simulink model "simcape_real_time_V3"  (R2022b)
settings: Solver=FixedStepAuto  StartTime=0.0  StopTime=100  FixedStep=0.002  RelTol=1e-3
undefined symbols (not defined in the file): drone_leg, K_LQR_GOC, pitch_init, roll_init, v_pitch_init, v_roll_init, v_x_init, v_y_init, v_yaw_init, v_z_init, X, x_init, Y, y_init, yaw_init, Z, z_init
libraries: sm_lib x70, nesl_utility x11, simulink x6
(part 4 of 4)

== matlab function simcape_real_time_V3/MATLAB Function ==
  data: T1 input; x2dot output; T2 input; T3 input; T4 input; roll input; pitch input; yaw input; roll_dot input; pitch_dot input; yaw_dot input; y2dot output; z2dot output; roll2dot output; pitch2dot output; yaw2dot output; HS_MSKK input; x_dot input; y_dot input; z_dot input
function [x2dot,y2dot,z2dot,roll2dot,pitch2dot,yaw2dot]= fcn(T1,T2,T3,T4,roll,pitch,yaw,roll_dot,pitch_dot,yaw_dot,HS_MSKK,x_dot,y_dot,z_dot)
    m = 1.7; %kg
    l = 0.25; %m
    % % b = 4.74E-5;
    % % d = 2.35E-7;
    g = 9.81; %ms2
    % % to = 0.05; %Nm
    Ix = 0.0030842; %kg.m2
    Iy = 0.0030842; %kg.m2
    Iz = 0.0032315; %kg.m2
    % Ir = 1E-4; %kg.m2
    U1 = T1+T2+T3+T4;
    U2 = l*(T2-T4);
    U3 = l*(T3-T1);
    U4 = T1-T2+T3-T4;

    x2dot=(U1*(sin(roll)*sin(yaw) + cos(roll)*cos(yaw)*sin(pitch)))/m;
    y2dot=-(U1*(cos(yaw)*sin(roll) - cos(roll)*sin(pitch)*sin(yaw)))/m;
    z2dot=(U1*cos(pitch)*cos(roll))/m - g;
    roll2dot=(Iy*pitch_dot*yaw_dot - Iz*pitch_dot*yaw_dot)/Ix + U2/Ix;
    pitch2dot=U3/Iy + (-Ix*roll_dot*yaw_dot + Iz*roll_dot*yaw_dot)/Iy;
    yaw2dot=U4/Iz + (Ix*pitch_dot*roll_dot - Iy*pitch_dot*roll_dot)/Iz;

% %% Gia lap ma sat theo cong thuc ma sat tuyen tinh voi he so cho truoc la
    FX_Friction     =  -  HS_MSKK * x_dot;
    FY_Friction     =  -  HS_MSKK * y_dot;
    FZ_Friction     =  -  HS_MSKK * z_dot;
    FR_Friction     =  -  HS_MSKK * roll_dot;
    FP_Friction     =  -  HS_MSKK * pitch_dot;
    FYaw_Friction   =  -  HS_MSKK * yaw_dot;
    FX_Limit        =     HS_MSKK /10;
    FY_Limit        =     HS_MSKK /10;
    FZ_Limit        =     HS_MSKK /10;
    FR_Limit        =     HS_MSKK /10;
    FP_Limit        =     HS_MSKK /10;
    FYaw_Limit      =     HS_MSKK /10;
    
    if(FX_Friction > FX_Limit)
        FX_Friction = FX_Limit;
    end
    if(FX_Friction < -FX_Limit)
        FX_Friction = -FX_Limit;
    end
    
    if(FY_Friction > FY_Limit)
        FY_Friction = FY_Limit;
    end
    if(FY_Friction < -FY_Limit)
        FY_Friction = -FY_Limit;
    end
    
    if(FZ_Friction > FZ_Limit)
        FZ_Friction = FZ_Limit;
    end
    if(FZ_Friction < -FZ_Limit)
        FZ_Friction = -FZ_Limit;
    end
    
    if(FR_Friction > FR_Limit)
        FR_Friction = FR_Limit;
    end
    if(FR_Friction < -FR_Limit)
        FR_Friction = -FR_Limit;
    end
    
    if(FP_Friction > FP_Limit)
        FP_Friction = FP_Limit;
    end
    if(FP_Friction < -FP_Limit)
        FP_Friction = -FP_Limit;
    end
    
    if(FYaw_Friction > FYaw_Limit)
        FYaw_Friction = FYaw_Limit;
    end
    if(FYaw_Friction < -FYaw_Limit)
        FYaw_Friction = -FYaw_Limit;
    end
    
    F_x2dot           = m*x2dot     - FX_Friction;
    if((m*x2dot)*(F_x2dot)<=0)
        F_x2dot     = m*x2dot;
    end
    F_y2dot           = m*y2dot     - FY_Friction;
    if((m*y2dot)*(F_y2dot)<=0)
        F_y2dot     = m*y2dot;
    end
    F_z2dot           = m*z2dot     - FZ_Friction;
    if((m*z2dot)*(F_z2dot)<=0)
        F_z2dot     = m*z2dot;
    end
    F_roll2dot        = m*roll2dot  - FR_Friction;
    if((m*roll2dot)*(F_roll2dot)<=0)
        F_roll2dot  = m*roll2dot;
    end
    F_pitch2dot       = m*pitch2dot - FP_Friction;
    if((m*pitch2dot)*(F_pitch2dot)<=0)
        F_pitch2dot = m*pitch2dot;
    end
    F_yaw2dot         = m*yaw2dot   - FYaw_Friction;
    if((m*yaw2dot)*(F_yaw2dot)<=0)
        F_yaw2dot   = m*yaw2dot;
    end

    x2dot           = F_x2dot/m;
    y2dot           = F_y2dot/m;
    z2dot           = F_z2dot/m;
    roll2dot        = F_roll2dot/m;
    pitch2dot       = F_pitch2dot/m;
    yaw2dot         = F_yaw2dot/m;
end
